simulink model "SimpleUnitTC2_SoftwareArch_vehicleDynamics_mapping"  (R2016b)
settings: Solver=FixedStepAuto  StartTime=0.0  StopTime=10.0  RelTol=1e-3
model workspace: external: MAT-File SimpleUnitTC2_SoftwareArch_vehicleDynamics_mapping.mat (data not in the file)
settings Model: Creator=NEATdemo  LastModifiedBy=NEATdemo

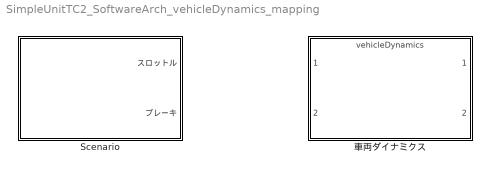
== system SimpleUnitTC2_SoftwareArch_vehicleDynamics_mapping ==
  Scenario : Subsystem
  車両ダイナミクス : ModelReference  ModelNameDialog=vehicleDynamics  SimulationMode=Normal  ModelReferenceVersion=1.8

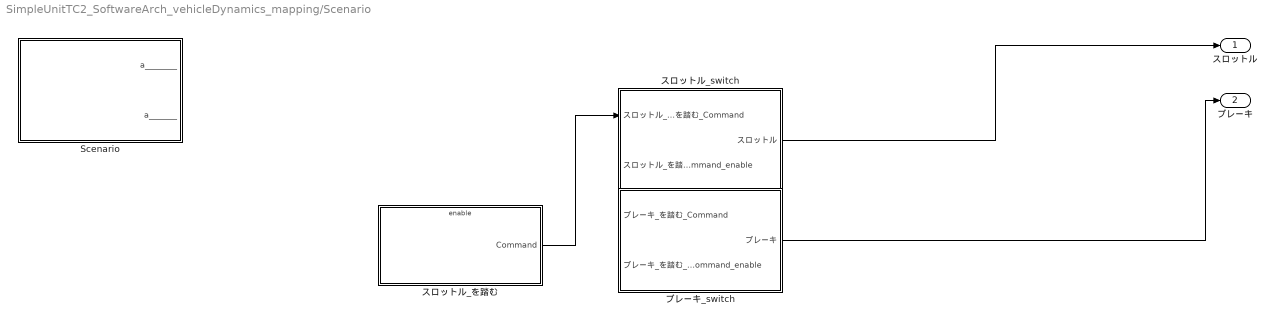
== system SimpleUnitTC2_SoftwareArch_vehicleDynamics_mapping/Scenario ==
  Scenario : Stateflow chart  TreatAsAtomicUnit=on
  スロットル_switch : Subsystem
  スロットル_を踏む : Subsystem
  ブレーキ_switch : Subsystem
  スロットル : Outport
  ブレーキ : Outport  Port=2
  wires:
  スロットル_switch/1(スロットル) -> スロットル/1
  ブレーキ_switch/1(ブレーキ) -> ブレーキ/1
  スロットル_を踏む/1(Command) -> スロットル_switch/1(スロットル_を踏む_Command)

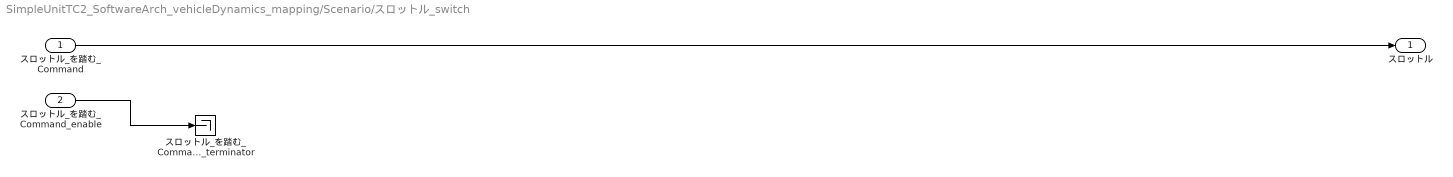
== system SimpleUnitTC2_SoftwareArch_vehicleDynamics_mapping/Scenario/スロットル_switch ==
  スロットル_を踏む_Command : Inport
  スロットル_を踏む_Command_enable : Inport  Port=2
  スロットル_を踏む_Command_terminator : Terminator
  スロットル : Outport
  wires:
  スロットル_を踏む_Command_enable/1 -> スロットル_を踏む_Command_terminator/1
  スロットル_を踏む_Command/1 -> スロットル/1

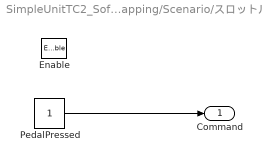
== system SimpleUnitTC2_SoftwareArch_vehicleDynamics_mapping/Scenario/スロットル_を踏む ==
  Enable : EnablePort
  PedalPressed : Constant
  Command : Outport  OutputWhenDisabled=reset  InitialOutput=0
  wires:
  PedalPressed/1 -> Command/1

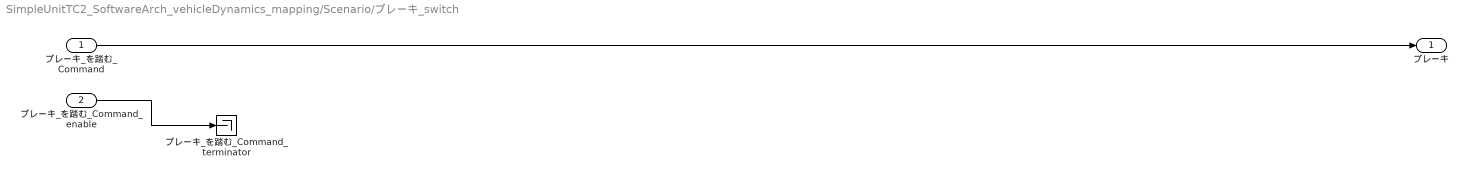
== system SimpleUnitTC2_SoftwareArch_vehicleDynamics_mapping/Scenario/ブレーキ_switch ==
  ブレーキ_を踏む_Command : Inport
  ブレーキ_を踏む_Command_enable : Inport  Port=2
  ブレーキ_を踏む_Command_terminator : Terminator
  ブレーキ : Outport
  wires:
  ブレーキ_を踏む_Command_enable/1 -> ブレーキ_を踏む_Command_terminator/1
  ブレーキ_を踏む_Command/1 -> ブレーキ/1

== stateflow chart SimpleUnitTC2_SoftwareArch_vehicleDynamics_mapping/Scenario/Scenario ==
  state Act_Subject_Step1
    entry: ブレーキ_を踏む = 0;
    entry: スロットル_を踏む = 1;
  (default) -> Act_Subject_Step1
  data: a________ output; a_______ output
